simulink model "GenerateImageDataOfParkingLot"  (R2023b)
settings: Solver=VariableStepAuto  StartTime=0.0  StopTime=60  RelTol=1e-3
undefined symbols (not defined in the file or in its folder): baseline, gray, refPosesT, refPosesX, refPosesY
libraries: sim3dautolib x60, sim3dcameralib x3, sim3dlib x1
(part 3 of 3)

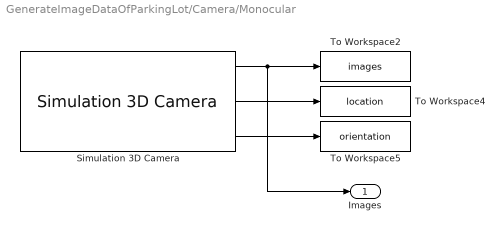
== system GenerateImageDataOfParkingLot/Camera/Monocular ==
  Simulation 3D Camera : sim3dcameralib/Simulation 3D Camera  Priority=1  sensorTag=Sim3dSensor7  sensorId=7  sensorName=Sim3dSensor7  vehTagList={'Scene Origin';'SimulinkVehicle1'}  vehTag=SimulinkVehicle1  mountLoc=Roof center  offsetFlag=off  tmountOffset=[0, 0, 0]  extTmount=off  rmountOffset=[0, 0, 0]  extRmount=off  FocalLength=focalLength  OpticalCenter=principalPoint  ImageSize=imageSize  RadialDistortion=[0, 0]  TangentialDistortion=[0, 0]  SensorSkew=0  DepthOutportEnabled=off  SemanticOutportEnabled=off  TransformOutportEnabled=on  SampleTime=-1  mountPoint=[0 0 1.55999994277954]  mountOrientation=[0 0 0]  aMode=3  ID=7
      settings: LibrarySourceBlock=drivingsim3d/Simulation 3D Camera
  To Workspace2 : ToWorkspace  VariableName=images  SaveFormat=Timeseries  SampleTime=-1
  To Workspace4 : ToWorkspace  VariableName=location  SaveFormat=Timeseries  SampleTime=-1
  To Workspace5 : ToWorkspace  VariableName=orientation  SaveFormat=Timeseries  SampleTime=-1
  Images : Outport
  wires:
  Simulation 3D Camera/2 -> To Workspace4/1
  Simulation 3D Camera/3 -> To Workspace5/1
  Simulation 3D Camera/1 -> Images/1, To Workspace2/1

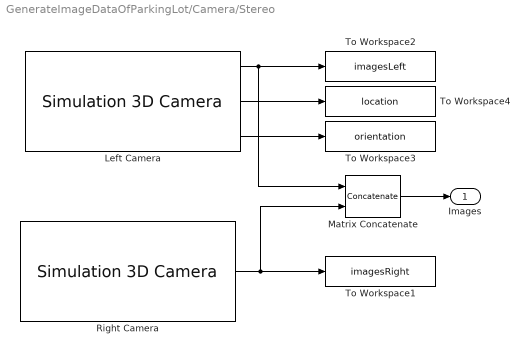
== system GenerateImageDataOfParkingLot/Camera/Stereo ==
  Left Camera : sim3dcameralib/Simulation 3D Camera  Priority=1  sensorTag=Sim3dSensor5  sensorId=5  sensorName=Sim3dSensor5  vehTagList={'Scene Origin';'SimulinkVehicle1'}  vehTag=SimulinkVehicle1  mountLoc=Roof center  offsetFlag=on  tmountOffset=[0, baseline/2, 0]  extTmount=off  rmountOffset=[0, 0, 0]  extRmount=off  FocalLength=focalLength  OpticalCenter=principalPoint  ImageSize=imageSize  RadialDistortion=[0, 0]  TangentialDistortion=[0, 0]  SensorSkew=0  DepthOutportEnabled=off  SemanticOutportEnabled=off  TransformOutportEnabled=on  SampleTime=-1  mountPoint=[0 -0.25 1.55999994277954]  mountOrientation=[0 0 0]  aMode=3  ID=5
      settings: LibrarySourceBlock=drivingsim3d/Simulation 3D Camera
  Matrix Concatenate : Concatenate  Mode=Multidimensional array
  Right Camera : sim3dcameralib/Simulation 3D Camera  Priority=1  sensorTag=Sim3dSensor6  sensorId=6  sensorName=Sim3dSensor6  vehTagList={'Scene Origin';'SimulinkVehicle1'}  vehTag=SimulinkVehicle1  mountLoc=Roof center  offsetFlag=on  tmountOffset=[0, -baseline/2, 0]  extTmount=off  rmountOffset=[0, 0, 0]  extRmount=off  FocalLength=focalLength  OpticalCenter=principalPoint  ImageSize=imageSize  RadialDistortion=[0, 0]  TangentialDistortion=[0, 0]  SensorSkew=0  DepthOutportEnabled=off  SemanticOutportEnabled=off  TransformOutportEnabled=off  SampleTime=-1  mountPoint=[0 0.25 1.55999994277954]  mountOrientation=[0 0 0]  aMode=3  ID=6
      settings: LibrarySourceBlock=drivingsim3d/Simulation 3D Camera
  To Workspace1 : ToWorkspace  VariableName=imagesRight  SaveFormat=Timeseries  SampleTime=-1
  To Workspace2 : ToWorkspace  VariableName=imagesLeft  SaveFormat=Timeseries  SampleTime=-1
  To Workspace3 : ToWorkspace  VariableName=orientation  SaveFormat=Timeseries  SampleTime=-1
  To Workspace4 : ToWorkspace  VariableName=location  SaveFormat=Timeseries  SampleTime=-1
  Images : Outport
  wires:
  Matrix Concatenate/1 -> Images/1
  Left Camera/2 -> To Workspace4/1
  Left Camera/1 -> To Workspace2/1, Matrix Concatenate/1
  Left Camera/3 -> To Workspace3/1
  Right Camera/1 -> To Workspace1/1, Matrix Concatenate/2
